simulink model "kopter_se_zavazim_Cascade_PID"  (R2024b)
settings: Solver=ode4  StartTime=0.0  StopTime=16  FixedStep=0.01  RelTol=1e-3
values from neighbouring files (symbols this model uses):
  A = 0.6081    [parametry_kopter_se_zavazim.m]
  b_moment = 3.6e-7    (= 3.6e-07)    [parametry_kopter_se_zavazim.m]
  d = 1    [parametry_kopter_se_zavazim.m]
  g = 9.81    [parametry_kopter_se_zavazim.m]
  Ip = m*d^2    (= 1)    [parametry_kopter_se_zavazim.m]
  Ixx = 0.0222    [parametry_kopter_se_zavazim.m]
  Iyy = 0.0222    [parametry_kopter_se_zavazim.m]
  Izz = 0.0429    [parametry_kopter_se_zavazim.m]
  k_thrust = 9.3e-6    (= 9.3e-06)    [parametry_kopter_se_zavazim.m]
  l = 0.2051    [parametry_kopter_se_zavazim.m]
  M = 2    [parametry_kopter_se_zavazim.m]
  m = 1    [parametry_kopter_se_zavazim.m]
  T = 0.8682    [parametry_kopter_se_zavazim.m]
  Us = [(M+m)*g; 0; 0; 0]    [parametry_kopter_se_zavazim.m]
  Xinit_ss = [Xinit_matrix; [0 0 0 0 0 0 0 0]']    [parametry_kopter_se_zavazim.m]
  Xs = [0;0;0; 0;0;0; 0;0; 0;0;0; 0;0;0; 0;0]    [parametry_kopter_se_zavazim.m]
undefined symbols (not defined in the file or in its folder): L, Us_p, Xs_p
libraries: simulink_extras x21, slpidlib x21, simulink x6
(part 2 of 5)

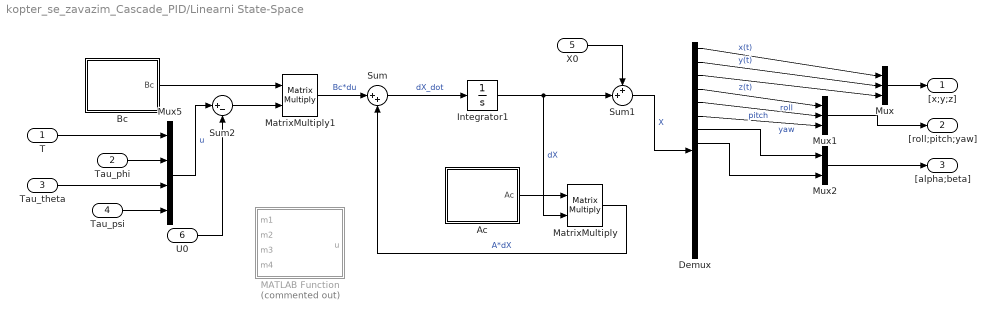
== system kopter_se_zavazim_Cascade_PID/Linearni State-Space ==
  T : Inport
  Tau_phi : Inport  Port=2
  Tau_theta : Inport  Port=3
  Tau_psi : Inport  Port=4
  X0 : Inport  Port=5
  U0 : Inport  Port=6
  Ac : MATLAB Function  TreatAsAtomicUnit=on
  Bc : MATLAB Function  TreatAsAtomicUnit=on
  Demux : Demux  Outputs=16
  Integrator1 : Integrator  InitialCondition=Xinit_ss - Xs
  MATLAB Function : MATLAB Function  Commented=on  TreatAsAtomicUnit=on
  MatrixMultiply : Product  Multiplication=Matrix(*)
  MatrixMultiply1 : Product  Multiplication=Matrix(*)
  Mux : Mux  Inputs=3
  Mux1 : Mux  Inputs=3
  Mux2 : Mux  Inputs=2
  Mux5 : Mux
  Sum : Sum  Inputs=|++
  Sum1 : Sum  Inputs=++|
  Sum2 : Sum  Inputs=|+-
  "[x;y;z]" : Outport
  "[roll;pitch;yaw]" : Outport  Port=2
  "[alpha;beta]" : Outport  Port=3
  wires:
  Ac/1(Ac) -> MatrixMultiply/1
  Integrator1/1 -> Sum1/2, MatrixMultiply/2  "dX"
  Demux/1 -> Mux/1  "x(t)"
  Demux/2 -> Mux/2  "y(t)"
  Demux/3 -> Mux/3  "z(t)"
  Mux/1 -> "[x;y;z]"/1
  Demux/4 -> Mux1/1  "roll"
  Demux/5 -> Mux1/2  "pitch"
  Demux/6 -> Mux1/3  "yaw"
  Mux1/1 -> "[roll;pitch;yaw]"/1
  Sum/1 -> Integrator1/1  "dX_dot"
  MatrixMultiply1/1 -> Sum/1  "Bc*du"
  MatrixMultiply/1 -> Sum/2  "A*dX"
  Bc/1(Bc) -> MatrixMultiply1/1
  Sum1/1 -> Demux/1  "X"
  Sum2/1 -> MatrixMultiply1/2
  Mux2/1 -> "[alpha;beta]"/1
  Demux/7 -> Mux2/1
  Demux/8 -> Mux2/2
  X0/1 -> Sum1/1
  U0/1 -> Sum2/2
  Mux5/1 -> Sum2/1  "u"
  Tau_psi/1 -> Mux5/4
  Tau_phi/1 -> Mux5/2
  Tau_theta/1 -> Mux5/3
  T/1 -> Mux5/1

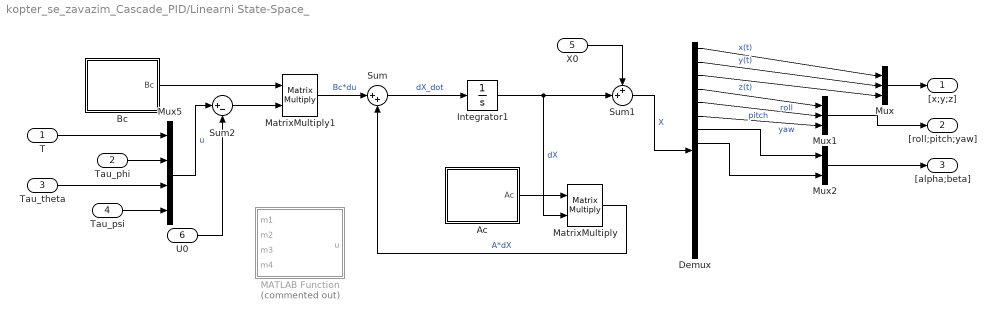
== system kopter_se_zavazim_Cascade_PID/Linearni State-Space_ ==
  T : Inport
  Tau_phi : Inport  Port=2
  Tau_theta : Inport  Port=3
  Tau_psi : Inport  Port=4
  X0 : Inport  Port=5
  U0 : Inport  Port=6
  Ac : MATLAB Function  TreatAsAtomicUnit=on
  Bc : MATLAB Function  TreatAsAtomicUnit=on
  Demux : Demux  Outputs=16
  Integrator1 : Integrator  InitialCondition=Xinit_ss
  MATLAB Function : MATLAB Function  Commented=on  TreatAsAtomicUnit=on
  MatrixMultiply : Product  Multiplication=Matrix(*)
  MatrixMultiply1 : Product  Multiplication=Matrix(*)
  Mux : Mux  Inputs=3
  Mux1 : Mux  Inputs=3
  Mux2 : Mux  Inputs=2
  Mux5 : Mux
  Sum : Sum  Inputs=|++
  Sum1 : Sum  Inputs=++|
  Sum2 : Sum  Inputs=|+-
  "[x;y;z]" : Outport
  "[roll;pitch;yaw]" : Outport  Port=2
  "[alpha;beta]" : Outport  Port=3
  wires:
  Ac/1(Ac) -> MatrixMultiply/1
  Integrator1/1 -> Sum1/2, MatrixMultiply/2  "dX"
  Demux/1 -> Mux/1  "x(t)"
  Demux/2 -> Mux/2  "y(t)"
  Demux/3 -> Mux/3  "z(t)"
  Mux/1 -> "[x;y;z]"/1
  Demux/4 -> Mux1/1  "roll"
  Demux/5 -> Mux1/2  "pitch"
  Demux/6 -> Mux1/3  "yaw"
  Mux1/1 -> "[roll;pitch;yaw]"/1
  Sum/1 -> Integrator1/1  "dX_dot"
  MatrixMultiply1/1 -> Sum/1  "Bc*du"
  MatrixMultiply/1 -> Sum/2  "A*dX"
  Bc/1(Bc) -> MatrixMultiply1/1
  Sum1/1 -> Demux/1  "X"
  Sum2/1 -> MatrixMultiply1/2
  Mux2/1 -> "[alpha;beta]"/1
  Demux/7 -> Mux2/1
  Demux/8 -> Mux2/2
  X0/1 -> Sum1/1
  U0/1 -> Sum2/2
  Mux5/1 -> Sum2/1  "u"
  Tau_psi/1 -> Mux5/4
  Tau_phi/1 -> Mux5/2
  Tau_theta/1 -> Mux5/3
  T/1 -> Mux5/1

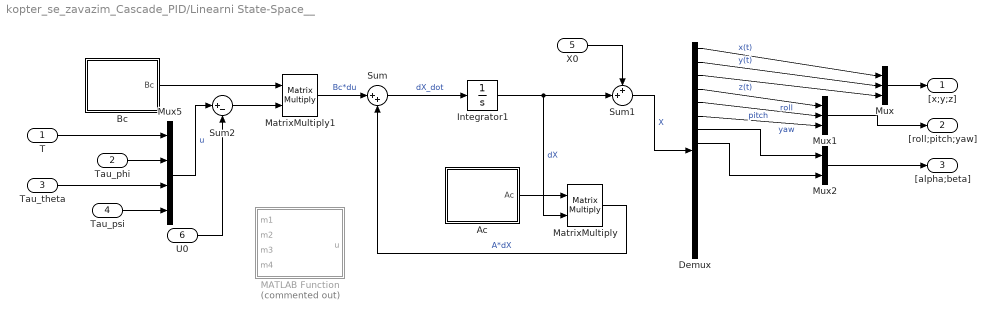
== system kopter_se_zavazim_Cascade_PID/Linearni State-Space__ ==
  T : Inport
  Tau_phi : Inport  Port=2
  Tau_theta : Inport  Port=3
  Tau_psi : Inport  Port=4
  X0 : Inport  Port=5
  U0 : Inport  Port=6
  Ac : MATLAB Function  TreatAsAtomicUnit=on
  Bc : MATLAB Function  TreatAsAtomicUnit=on
  Demux : Demux  Outputs=16
  Integrator1 : Integrator  InitialCondition=Xinit_ss
  MATLAB Function : MATLAB Function  Commented=on  TreatAsAtomicUnit=on
  MatrixMultiply : Product  Multiplication=Matrix(*)
  MatrixMultiply1 : Product  Multiplication=Matrix(*)
  Mux : Mux  Inputs=3
  Mux1 : Mux  Inputs=3
  Mux2 : Mux  Inputs=2
  Mux5 : Mux
  Sum : Sum  Inputs=|++
  Sum1 : Sum  Inputs=++|
  Sum2 : Sum  Inputs=|+-
  "[x;y;z]" : Outport
  "[roll;pitch;yaw]" : Outport  Port=2
  "[alpha;beta]" : Outport  Port=3
  wires:
  Ac/1(Ac) -> MatrixMultiply/1
  Integrator1/1 -> Sum1/2, MatrixMultiply/2  "dX"
  Demux/1 -> Mux/1  "x(t)"
  Demux/2 -> Mux/2  "y(t)"
  Demux/3 -> Mux/3  "z(t)"
  Mux/1 -> "[x;y;z]"/1
  Demux/4 -> Mux1/1  "roll"
  Demux/5 -> Mux1/2  "pitch"
  Demux/6 -> Mux1/3  "yaw"
  Mux1/1 -> "[roll;pitch;yaw]"/1
  Sum/1 -> Integrator1/1  "dX_dot"
  MatrixMultiply1/1 -> Sum/1  "Bc*du"
  MatrixMultiply/1 -> Sum/2  "A*dX"
  Bc/1(Bc) -> MatrixMultiply1/1
  Sum1/1 -> Demux/1  "X"
  Sum2/1 -> MatrixMultiply1/2
  Mux2/1 -> "[alpha;beta]"/1
  Demux/7 -> Mux2/1
  Demux/8 -> Mux2/2
  X0/1 -> Sum1/1
  U0/1 -> Sum2/2
  Mux5/1 -> Sum2/1  "u"
  Tau_psi/1 -> Mux5/4
  Tau_phi/1 -> Mux5/2
  Tau_theta/1 -> Mux5/3
  T/1 -> Mux5/1

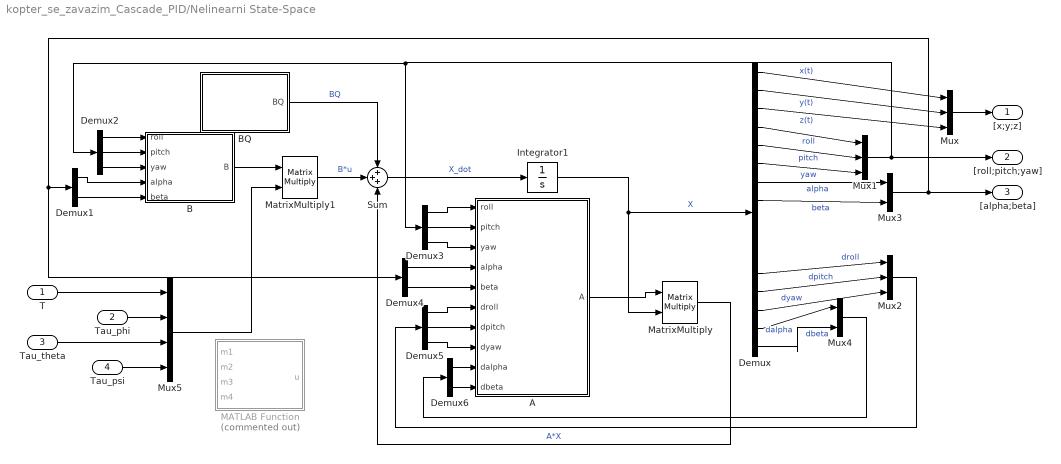
== system kopter_se_zavazim_Cascade_PID/Nelinearni State-Space ==
  T : Inport
  Tau_phi : Inport  Port=2
  Tau_theta : Inport  Port=3
  Tau_psi : Inport  Port=4
  A : MATLAB Function  TreatAsAtomicUnit=on
  B : MATLAB Function  TreatAsAtomicUnit=on
  BQ : MATLAB Function  TreatAsAtomicUnit=on
  Demux : Demux  Outputs=16
  Demux1 : Demux  Outputs=2
  Demux2 : Demux  Outputs=3
  Demux3 : Demux  Outputs=3
  Demux4 : Demux  Outputs=2
  Demux5 : Demux  Outputs=3
  Demux6 : Demux  Outputs=2
  Integrator1 : Integrator  InitialCondition=Xinit_ss
  MATLAB Function : MATLAB Function  Commented=on  TreatAsAtomicUnit=on
  MatrixMultiply : Product  Multiplication=Matrix(*)
  MatrixMultiply1 : Product  Multiplication=Matrix(*)
  Mux : Mux  Inputs=3
  Mux1 : Mux  Inputs=3
  Mux2 : Mux  Inputs=3
  Mux3 : Mux  Inputs=2
  Mux4 : Mux  Inputs=2
  Mux5 : Mux
  Sum : Sum  Inputs=+++
  "[x;y;z]" : Outport
  "[roll;pitch;yaw]" : Outport  Port=2
  "[alpha;beta]" : Outport  Port=3
  wires:
  A/1(A) -> MatrixMultiply/1
  Integrator1/1 -> MatrixMultiply/2, Demux/1  "X"
  Demux/1 -> Mux/1  "x(t)"
  Demux/2 -> Mux/2  "y(t)"
  Demux/3 -> Mux/3  "z(t)"
  Mux/1 -> "[x;y;z]"/1
  Demux/4 -> Mux1/1  "roll"
  Demux/5 -> Mux1/2  "pitch"
  Demux/6 -> Mux1/3  "yaw"
  Mux1/1 -> Demux2/1, Demux3/1, "[roll;pitch;yaw]"/1
  Demux/12 -> Mux2/1  "droll"
  Demux/13 -> Mux2/2  "dpitch"
  Demux/14 -> Mux2/3  "dyaw"
  Demux2/1 -> B/1(roll)
  Demux2/2 -> B/2(pitch)
  Demux2/3 -> B/3(yaw)
  Demux3/2 -> A/2(pitch)
  Demux3/1 -> A/1(roll)
  Demux3/3 -> A/3(yaw)
  Demux5/2 -> A/7(dpitch)
  Demux5/1 -> A/6(droll)
  Demux5/3 -> A/8(dyaw)
  Sum/1 -> Integrator1/1  "X_dot"
  BQ/1(BQ) -> Sum/1  "BQ"
  MatrixMultiply1/1 -> Sum/2  "B*u"
  B/1(B) -> MatrixMultiply1/1
  MatrixMultiply/1 -> Sum/3  "A*X"
  Mux2/1 -> Demux5/1
  Demux/7 -> Mux3/1  "alpha"
  Demux/8 -> Mux3/2  "beta"
  Mux3/1 -> Demux4/1, Demux1/1, "[alpha;beta]"/1
  Demux1/2 -> B/5(beta)
  Demux1/1 -> B/4(alpha)
  Demux4/2 -> A/5(beta)
  Demux4/1 -> A/4(alpha)
  Demux/15 -> Mux4/1  "dalpha"
  Demux/16 -> Mux4/2  "dbeta"
  Demux6/1 -> A/9(dalpha)
  Demux6/2 -> A/10(dbeta)
  Mux4/1 -> Demux6/1
  Tau_theta/1 -> Mux5/3
  Tau_psi/1 -> Mux5/4
  Tau_phi/1 -> Mux5/2
  Mux5/1 -> MatrixMultiply1/2
  T/1 -> Mux5/1

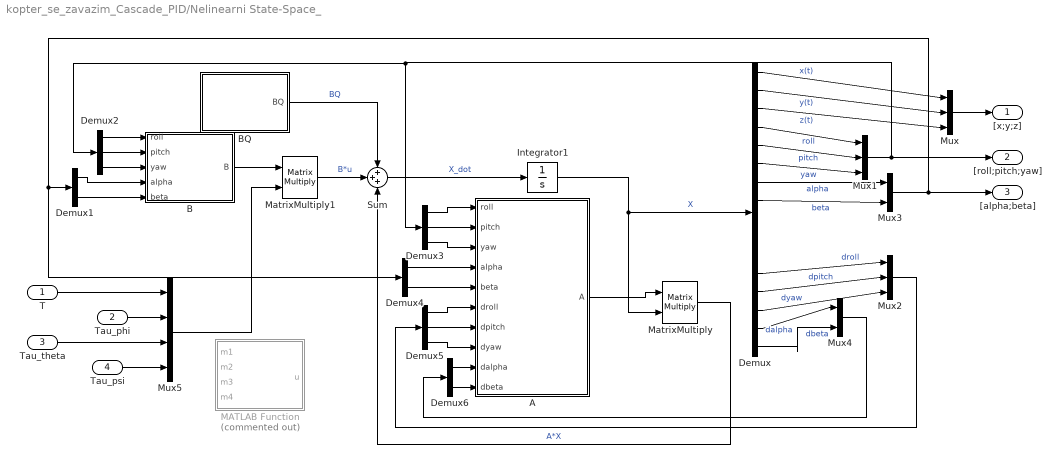
== system kopter_se_zavazim_Cascade_PID/Nelinearni State-Space_ ==
  T : Inport
  Tau_phi : Inport  Port=2
  Tau_theta : Inport  Port=3
  Tau_psi : Inport  Port=4
  A : MATLAB Function  TreatAsAtomicUnit=on
  B : MATLAB Function  TreatAsAtomicUnit=on
  BQ : MATLAB Function  TreatAsAtomicUnit=on
  Demux : Demux  Outputs=16
  Demux1 : Demux  Outputs=2
  Demux2 : Demux  Outputs=3
  Demux3 : Demux  Outputs=3
  Demux4 : Demux  Outputs=2
  Demux5 : Demux  Outputs=3
  Demux6 : Demux  Outputs=2
  Integrator1 : Integrator  InitialCondition=Xinit_ss
  MATLAB Function : MATLAB Function  Commented=on  TreatAsAtomicUnit=on
  MatrixMultiply : Product  Multiplication=Matrix(*)
  MatrixMultiply1 : Product  Multiplication=Matrix(*)
  Mux : Mux  Inputs=3
  Mux1 : Mux  Inputs=3
  Mux2 : Mux  Inputs=3
  Mux3 : Mux  Inputs=2
  Mux4 : Mux  Inputs=2
  Mux5 : Mux
  Sum : Sum  Inputs=+++
  "[x;y;z]" : Outport
  "[roll;pitch;yaw]" : Outport  Port=2
  "[alpha;beta]" : Outport  Port=3
  wires:
  A/1(A) -> MatrixMultiply/1
  Integrator1/1 -> MatrixMultiply/2, Demux/1  "X"
  Demux/1 -> Mux/1  "x(t)"
  Demux/2 -> Mux/2  "y(t)"
  Demux/3 -> Mux/3  "z(t)"
  Mux/1 -> "[x;y;z]"/1
  Demux/4 -> Mux1/1  "roll"
  Demux/5 -> Mux1/2  "pitch"
  Demux/6 -> Mux1/3  "yaw"
  Mux1/1 -> Demux2/1, Demux3/1, "[roll;pitch;yaw]"/1
  Demux/12 -> Mux2/1  "droll"
  Demux/13 -> Mux2/2  "dpitch"
  Demux/14 -> Mux2/3  "dyaw"
  Demux2/1 -> B/1(roll)
  Demux2/2 -> B/2(pitch)
  Demux2/3 -> B/3(yaw)
  Demux3/2 -> A/2(pitch)
  Demux3/1 -> A/1(roll)
  Demux3/3 -> A/3(yaw)
  Demux5/2 -> A/7(dpitch)
  Demux5/1 -> A/6(droll)
  Demux5/3 -> A/8(dyaw)
  Sum/1 -> Integrator1/1  "X_dot"
  BQ/1(BQ) -> Sum/1  "BQ"
  MatrixMultiply1/1 -> Sum/2  "B*u"
  B/1(B) -> MatrixMultiply1/1
  MatrixMultiply/1 -> Sum/3  "A*X"
  Mux2/1 -> Demux5/1
  Demux/7 -> Mux3/1  "alpha"
  Demux/8 -> Mux3/2  "beta"
  Mux3/1 -> Demux4/1, Demux1/1, "[alpha;beta]"/1
  Demux1/2 -> B/5(beta)
  Demux1/1 -> B/4(alpha)
  Demux4/2 -> A/5(beta)
  Demux4/1 -> A/4(alpha)
  Demux/15 -> Mux4/1  "dalpha"
  Demux/16 -> Mux4/2  "dbeta"
  Demux6/1 -> A/9(dalpha)
  Demux6/2 -> A/10(dbeta)
  Mux4/1 -> Demux6/1
  Tau_theta/1 -> Mux5/3
  Tau_psi/1 -> Mux5/4
  Tau_phi/1 -> Mux5/2
  Mux5/1 -> MatrixMultiply1/2
  T/1 -> Mux5/1

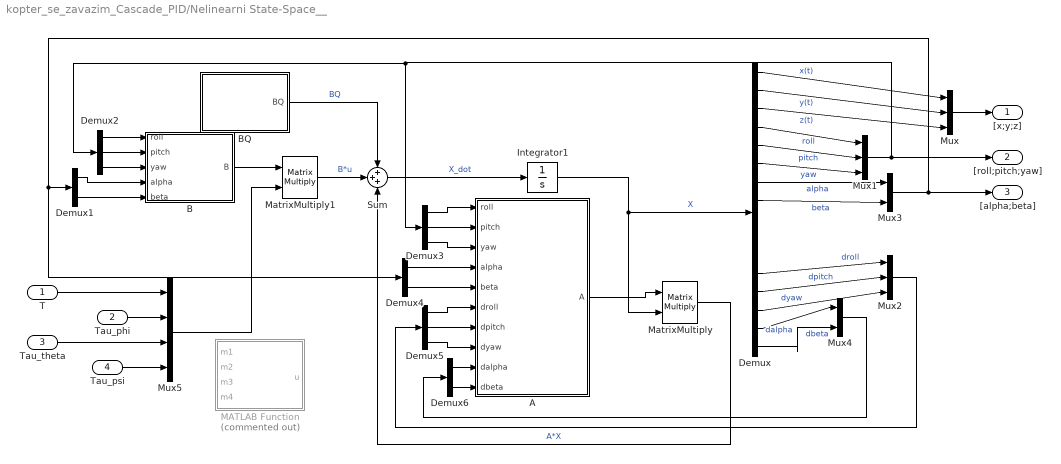
== system kopter_se_zavazim_Cascade_PID/Nelinearni State-Space__ ==
  T : Inport
  Tau_phi : Inport  Port=2
  Tau_theta : Inport  Port=3
  Tau_psi : Inport  Port=4
  A : MATLAB Function  TreatAsAtomicUnit=on
  B : MATLAB Function  TreatAsAtomicUnit=on
  BQ : MATLAB Function  TreatAsAtomicUnit=on
  Demux : Demux  Outputs=16
  Demux1 : Demux  Outputs=2
  Demux2 : Demux  Outputs=3
  Demux3 : Demux  Outputs=3
  Demux4 : Demux  Outputs=2
  Demux5 : Demux  Outputs=3
  Demux6 : Demux  Outputs=2
  Integrator1 : Integrator  InitialCondition=Xinit_ss
  MATLAB Function : MATLAB Function  Commented=on  TreatAsAtomicUnit=on
  MatrixMultiply : Product  Multiplication=Matrix(*)
  MatrixMultiply1 : Product  Multiplication=Matrix(*)
  Mux : Mux  Inputs=3
  Mux1 : Mux  Inputs=3
  Mux2 : Mux  Inputs=3
  Mux3 : Mux  Inputs=2
  Mux4 : Mux  Inputs=2
  Mux5 : Mux
  Sum : Sum  Inputs=+++
  "[x;y;z]" : Outport
  "[roll;pitch;yaw]" : Outport  Port=2
  "[alpha;beta]" : Outport  Port=3
  wires:
  A/1(A) -> MatrixMultiply/1
  Integrator1/1 -> MatrixMultiply/2, Demux/1  "X"
  Demux/1 -> Mux/1  "x(t)"
  Demux/2 -> Mux/2  "y(t)"
  Demux/3 -> Mux/3  "z(t)"
  Mux/1 -> "[x;y;z]"/1
  Demux/4 -> Mux1/1  "roll"
  Demux/5 -> Mux1/2  "pitch"
  Demux/6 -> Mux1/3  "yaw"
  Mux1/1 -> Demux2/1, Demux3/1, "[roll;pitch;yaw]"/1
  Demux/12 -> Mux2/1  "droll"
  Demux/13 -> Mux2/2  "dpitch"
  Demux/14 -> Mux2/3  "dyaw"
  Demux2/1 -> B/1(roll)
  Demux2/2 -> B/2(pitch)
  Demux2/3 -> B/3(yaw)
  Demux3/2 -> A/2(pitch)
  Demux3/1 -> A/1(roll)
  Demux3/3 -> A/3(yaw)
  Demux5/2 -> A/7(dpitch)
  Demux5/1 -> A/6(droll)
  Demux5/3 -> A/8(dyaw)
  Sum/1 -> Integrator1/1  "X_dot"
  BQ/1(BQ) -> Sum/1  "BQ"
  MatrixMultiply1/1 -> Sum/2  "B*u"
  B/1(B) -> MatrixMultiply1/1
  MatrixMultiply/1 -> Sum/3  "A*X"
  Mux2/1 -> Demux5/1
  Demux/7 -> Mux3/1  "alpha"
  Demux/8 -> Mux3/2  "beta"
  Mux3/1 -> Demux4/1, Demux1/1, "[alpha;beta]"/1
  Demux1/2 -> B/5(beta)
  Demux1/1 -> B/4(alpha)
  Demux4/2 -> A/5(beta)
  Demux4/1 -> A/4(alpha)
  Demux/15 -> Mux4/1  "dalpha"
  Demux/16 -> Mux4/2  "dbeta"
  Demux6/1 -> A/9(dalpha)
  Demux6/2 -> A/10(dbeta)
  Mux4/1 -> Demux6/1
  Tau_theta/1 -> Mux5/3
  Tau_psi/1 -> Mux5/4
  Tau_phi/1 -> Mux5/2
  Mux5/1 -> MatrixMultiply1/2
  T/1 -> Mux5/1

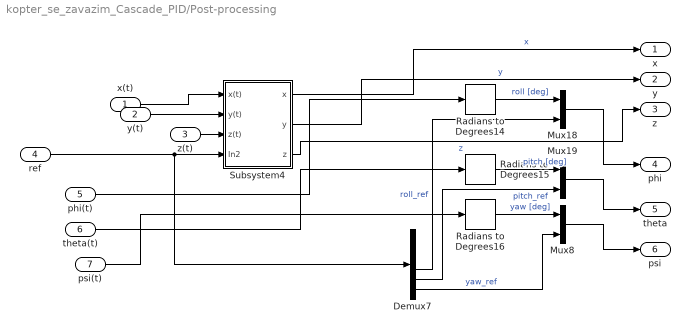
== system kopter_se_zavazim_Cascade_PID/Post-processing ==
  x(t) : Inport
  y(t) : Inport  Port=2
  z(t) : Inport  Port=3
  ref : Inport  Port=4
  phi(t) : Inport  Port=5
  theta(t) : Inport  Port=6
  psi(t) : Inport  Port=7
  Demux7 : Demux  Outputs=6
  Mux18 : Mux  Inputs=2
  Mux19 : Mux  Inputs=2
  Mux8 : Mux  Inputs=2
  Radians to Degrees14 : simulink_extras/Transformations/Radians to Degrees
  Radians to Degrees15 : simulink_extras/Transformations/Radians to Degrees
  Radians to Degrees16 : simulink_extras/Transformations/Radians to Degrees
  Subsystem4 : Subsystem
  x : Outport
  y : Outport  Port=2
  z : Outport  Port=3
  phi : Outport  Port=4
  theta : Outport  Port=5
  psi : Outport  Port=6
  wires:
  Radians to Degrees16/1 -> Mux8/1  "yaw [deg]"
  ref/1 -> Subsystem4/4(In2), Demux7/1
  Demux7/6 -> Mux8/2  "yaw_ref"
  theta(t)/1 -> Radians to Degrees15/1
  Demux7/4 -> Mux18/2  "roll_ref"
  Demux7/5 -> Mux19/2  "pitch_ref"
  Mux18/1 -> phi/1
  Subsystem4/3(z) -> z/1  "z"
  Radians to Degrees14/1 -> Mux18/1  "roll [deg]"
  Radians to Degrees15/1 -> Mux19/1  "pitch [deg]"
  Subsystem4/2(y) -> y/1  "y"
  x(t)/1 -> Subsystem4/1(x(t))
  y(t)/1 -> Subsystem4/2(y(t))
  psi(t)/1 -> Radians to Degrees16/1
  phi(t)/1 -> Radians to Degrees14/1
  Subsystem4/1(x) -> x/1  "x"
  Mux8/1 -> psi/1
  z(t)/1 -> Subsystem4/3(z(t))
  Mux19/1 -> theta/1

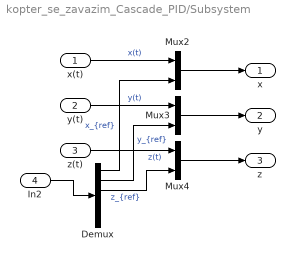
== system kopter_se_zavazim_Cascade_PID/Subsystem ==
  x(t) : Inport
  y(t) : Inport  Port=2
  z(t) : Inport  Port=3
  In2 : Inport  Port=4
  Demux : Demux  Outputs=6
  Mux2 : Mux  Inputs=2
  Mux3 : Mux  Inputs=2
  Mux4 : Mux  Inputs=2
  x : Outport
  y : Outport  Port=2
  z : Outport  Port=3
  wires:
  Demux/2 -> Mux3/2  "y_{ref}"
  Mux4/1 -> z/1
  y(t)/1 -> Mux3/1  "y(t)"
  Mux3/1 -> y/1
  Demux/1 -> Mux2/2  "x_{ref}"
  Demux/3 -> Mux4/2  "z_{ref}"
  Mux2/1 -> x/1
  In2/1 -> Demux/1
  x(t)/1 -> Mux2/1  "x(t)"
  z(t)/1 -> Mux4/1  "z(t)"

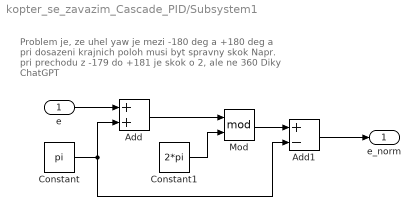
== system kopter_se_zavazim_Cascade_PID/Subsystem1 ==
  note: Problem je, ze uhel yaw je mezi -180 deg a +180 deg
      | a pri dosazeni krajnich poloh musi byt spravny skok
      | Napr. pri prechodu z -179 do +181 je skok o 2, ale ne 360
      | Diky ChatGPT
  e : Inport
  Add : Sum
  Add1 : Sum  Inputs=+-
  Constant : Constant  Value=pi
  Constant1 : Constant  Value=2*pi
  Mod : Math  Operator=mod
  e_norm : Outport
  wires:
  e/1 -> Add/1
  Add/1 -> Mod/1
  Constant/1 -> Add1/2, Add/2
  Constant1/1 -> Mod/2
  Mod/1 -> Add1/1
  Add1/1 -> e_norm/1

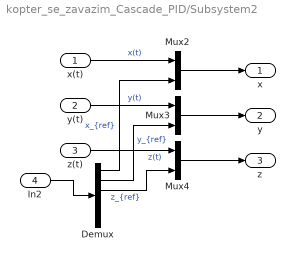
== system kopter_se_zavazim_Cascade_PID/Subsystem2 ==
  x(t) : Inport
  y(t) : Inport  Port=2
  z(t) : Inport  Port=3
  In2 : Inport  Port=4
  Demux : Demux  Outputs=6
  Mux2 : Mux  Inputs=2
  Mux3 : Mux  Inputs=2
  Mux4 : Mux  Inputs=2
  x : Outport
  y : Outport  Port=2
  z : Outport  Port=3
  wires:
  Demux/2 -> Mux3/2  "y_{ref}"
  Mux4/1 -> z/1
  y(t)/1 -> Mux3/1  "y(t)"
  Mux3/1 -> y/1
  Demux/1 -> Mux2/2  "x_{ref}"
  Demux/3 -> Mux4/2  "z_{ref}"
  Mux2/1 -> x/1
  In2/1 -> Demux/1
  x(t)/1 -> Mux2/1  "x(t)"
  z(t)/1 -> Mux4/1  "z(t)"

== system kopter_se_zavazim_Cascade_PID/Subsystem3 ==
  note: Problem je, ze uhel yaw je mezi -180 deg a +180 deg
      | a pri dosazeni krajnich poloh musi byt spravny skok
      | Napr. pri prechodu z -179 do +181 je skok o 2, ale ne 360
      | Diky ChatGPT
  e : Inport
  Add : Sum
  Add1 : Sum  Inputs=+-
  Constant : Constant  Value=pi
  Constant1 : Constant  Value=2*pi
  Mod : Math  Operator=mod
  e_norm : Outport
  wires:
  e/1 -> Add/1
  Add/1 -> Mod/1
  Constant/1 -> Add1/2, Add/2
  Constant1/1 -> Mod/2
  Mod/1 -> Add1/1
  Add1/1 -> e_norm/1

== system kopter_se_zavazim_Cascade_PID/[-pi; pi] calc ==
  note: Problem je, ze uhel yaw je mezi -180 deg a +180 deg
      | a pri dosazeni krajnich poloh musi byt spravny skok
      | Napr. pri prechodu z -179 do +181 je skok o 2, ale ne 360
      | Diky ChatGPT
  e : Inport
  Add : Sum
  Add1 : Sum  Inputs=+-
  Constant : Constant  Value=pi
  Constant1 : Constant  Value=2*pi
  Mod : Math  Operator=mod
  e_norm : Outport
  wires:
  e/1 -> Add/1
  Add/1 -> Mod/1
  Constant/1 -> Add1/2, Add/2
  Constant1/1 -> Mod/2
  Mod/1 -> Add1/1
  Add1/1 -> e_norm/1

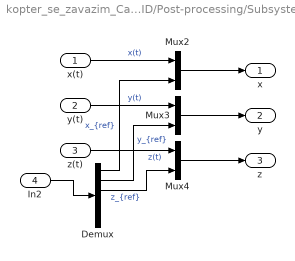
== system kopter_se_zavazim_Cascade_PID/Post-processing/Subsystem4 ==
  x(t) : Inport
  y(t) : Inport  Port=2
  z(t) : Inport  Port=3
  In2 : Inport  Port=4
  Demux : Demux  Outputs=6
  Mux2 : Mux  Inputs=2
  Mux3 : Mux  Inputs=2
  Mux4 : Mux  Inputs=2
  x : Outport
  y : Outport  Port=2
  z : Outport  Port=3
  wires:
  Demux/2 -> Mux3/2  "y_{ref}"
  Mux4/1 -> z/1
  y(t)/1 -> Mux3/1  "y(t)"
  Mux3/1 -> y/1
  Demux/1 -> Mux2/2  "x_{ref}"
  Demux/3 -> Mux4/2  "z_{ref}"
  Mux2/1 -> x/1
  In2/1 -> Demux/1
  x(t)/1 -> Mux2/1  "x(t)"
  z(t)/1 -> Mux4/1  "z(t)"

== matlab function kopter_se_zavazim_Cascade_PID/(rad//s)^2 na sily ==
  data: u output; U1 input; U2 input; U3 input; U4 input; k_thrust parameter; b_moment parameter; l parameter
function u = fcn(U1, U2, U3, U4, k_thrust, b_moment, l)

T = k_thrust*(U1+U2+U3+U4);
Tau_roll = k_thrust*l*(U1+U4-U2-U3);
Tau_pitch = k_thrust*l*(U3+U4-U1-U2);
Tau_yaw = b_moment*(U1+U3-U2-U4);

u = [T; Tau_roll; Tau_pitch; Tau_yaw];

== matlab function kopter_se_zavazim_Cascade_PID/Linearni State-Space_/Bc ==
  data: M parameter; Bc output; Ixx parameter; Iyy parameter; Izz parameter; m parameter
function Bc = fcn(M, Ixx, Iyy, Izz, m)
% Matice Bc linearizovana

Bc = [
        0,     0,     0,     0;
        0,     0,     0,     0;
        0,     0,     0,     0;
        0,     0,     0,     0;
        0,     0,     0,     0;
        0,     0,     0,     0;
        0,     0,     0,     0;
        0,     0,     0,     0;
        0,     0,     0,     0;
        0,     0,     0,     0;
1/(M + m),     0,     0,     0;
        0, 1/Ixx,     0,     0;
        0,     0, 1/Iyy,     0;
        0,     0,     0, 1/Izz;
        0,     0,     0,     0;
        0,     0,     0,     0];

== matlab function kopter_se_zavazim_Cascade_PID/Linearni State-Space_/MATLAB Function ==
  data: u output; m1 input; m2 input; m3 input; m4 input; k_thrust parameter; b_moment parameter; l parameter
function u = fcn(m1, m2, m3, m4, k_thrust, b_moment, l)

Thrust = k_thrust*(m1^2 + m2^2 + m3^2 + m4^2);
Tau_roll = l*k_thrust*(m1^2 + m4^2 - m2^2 - m3^2);
Tau_pitch = l*k_thrust*(m4^2 + m3^2 - m1^2 - m2^2);
Tau_yaw = b_moment*(m1^2 + m3^2 - m2^2 - m4^2);

u = [Thrust; Tau_roll; Tau_pitch; Tau_yaw];

== matlab function kopter_se_zavazim_Cascade_PID/Fi do [T; moments]_ ==
  data: F1 input; u output; F2 input; F3 input; F4 input; k_thrust parameter; b_moment parameter; l parameter
function u = fcn(F1, F2, F3, F4, k_thrust, b_moment, l)
% Dle X tvaru kvadrokoptery dopocitavam 
% celkovou tahovou silu T a tri momenty
T = F1+F2+F3+F4;
Tau_phi = l*(F1+F4-F2-F3);
Tau_theta = l*(F3+F4-F1-F2);
Tau_psi = b_moment/k_thrust*(F1-F2+F3-F4);

u = [T; Tau_phi; Tau_theta; Tau_psi];

== matlab function kopter_se_zavazim_Cascade_PID/Fi to [T; moments] ==
  data: F1 input; inputs output; F2 input; F3 input; F4 input; k_thrust parameter; b_moment parameter; l parameter
function inputs = fcn(F1, F2, F3, F4, k_thrust, b_moment, l)
% Dle X tvaru kvadrokoptery dopocitavam 
% celkovou tahovou silu T a tri momenty
T = F1+F2+F3+F4;
Tau_phi = l*(F1+F4-F2-F3);
Tau_theta = l*(F3+F4-F1-F2);
Tau_psi = b_moment/k_thrust*(F1-F2+F3-F4);

inputs = [T; Tau_phi; Tau_theta; Tau_psi];

== matlab function kopter_se_zavazim_Cascade_PID/Nelinearni State-Space_/A ==
  data: roll input; A output; pitch input; yaw input; alpha input; beta input; droll input; dpitch input; dyaw input; dalpha input; dbeta input; Ixx parameter; Iyy parameter; Izz parameter; M parameter; Ip parameter; d parameter; m parameter
function A = fcn(roll, pitch, yaw, alpha, beta, droll, dpitch, dyaw, dalpha, dbeta, Ixx, Iyy, Izz, M, Ip, d, m)
% Matice dynamiky A

phi_t = roll;
theta_t = pitch;
psi_t = yaw;

alpha_t = alpha;
beta_t = beta;

phi_dot_t = droll;
theta_dot_t = dpitch;
psi_dot_t = dyaw;

alpha_dot_t = dalpha;
beta_dot_t = dbeta;

A = [ 
0, 0, 0, 0, 0, 0, 0, 0, 1, 0, 0,                                                                                                                                                                                                                                                                                                                                                                                                                                                                                                           0,                                                                                                                                                                                                                                                                                                                                                                                                                                                                                                                                                                                                                                                                                                                              0,                                                                                                                                                                                            0,                                                          0,                                                  0;
0, 0, 0, 0, 0, 0, 0, 0, 0, 1, 0,                                                                                                                                                                                                                                                                                                                                                                                                                                                                                                           0,                                                                                                                                                                                                                                                                                                                                                                                                                                                                                                                                                                                                                                                                                                                              0,                                                                                                                                                                                            0,                                                          0,                                                  0;
0, 0, 0, 0, 0, 0, 0, 0, 0, 0, 1,                                                                                                                                                                                                                                                                                                                                                                                                                                                                                                           0,                                                                                                                                                                                                                                                                                                                                                                                                                                                                                                                                                                                                                                                                                                                              0,                                                                                                                                                                                            0,                                                          0,                                                  0;
0, 0, 0, 0, 0, 0, 0, 0, 0, 0, 0,                                                                                                                                                                                                                                                                                                                                                                                                                                                                                                           1,                                                                                                                                                                                                                                                                                                                                                                                                                                                                                                                                                                                                                                                                                                                              0,                                                                                                                                                                                            0,                                                          0,                                                  0;
0, 0, 0, 0, 0, 0, 0, 0, 0, 0, 0,                                                                                                                                                                                                                                                                                                                                                                                                                                                                                                           0,                                                                                                                                                                                                                                                                                                                                                                                                                                                                                                                                                                                                                                                                                                                              1,                                                                                                                                                                                            0,                                                          0,                                                  0;
0, 0, 0, 0, 0, 0, 0, 0, 0, 0, 0,                                                                                                                                                                                                                                                                                                                                                                                                                                                                                                           0,                                                                                                                                                                                                                                                                                                                                                                                                                                                                                                                                                                                                                                                                                                                              0,                                                                                                                                                                                            1,                                                          0,                                                  0;
0, 0, 0, 0, 0, 0, 0, 0, 0, 0, 0,                                                                                                                                                                                                                                                                                                                                                                                                                                                                                                           0,                                                                                                                                                                                                                                                                                                                                                                                                                                                                                                                                                                                                                                                                                                                              0,                                                                                                                                                                                            0,                                                          1,                                                  0;
0, 0, 0, 0, 0, 0, 0, 0, 0, 0, 0,                                                                                                                                                                                                                                                                                                                                                                                                                                                                                                           0,                                                                                                                                                                                                                                                                                                                                                                                                                                                                                                                                                                                                                                                                                                                              0,                                                                                                                                                                                            0,                                                          0,                                                  1;
0, 0, 0, 0, 0, 0, 0, 0, 0, 0, 0,                                                                                                                                                                                                                                                                                                                                                                                                                                                                                                           0,                                                                                                                                                                                                                                                                                                                                                                                                                                                                                                                                                                                                                                                                                                                              0,                                                                                                                                                                                            0,       (alpha_dot_t*d*m*cos(beta_t)^3*sin(alpha_t))/(M + m),  (beta_dot_t*d*m*cos(beta_t)*sin(alpha_t))/(M + m);
0, 0, 0, 0, 0, 0, 0, 0, 0, 0, 0,                                                                                                                                                                                                                                                                                                                                                                                                                                                                                                           0,                                                                                                                                                                                                                                                                                                                                                                                                                                                                                                                                                                                                                                                                                                                              0,                                                                                                                                                                                            0, -(alpha_dot_t*d*m*sin(beta_t)*(sin(beta_t)^2 - 1))/(M + m),               (beta_dot_t*d*m*sin(beta_t))/(M + m);
0, 0, 0, 0, 0, 0, 0, 0, 0, 0, 0,                                                                                                                                                                                                                                                                                                                                                                                                                                                                                                           0,                                                                                                                                                                                                                                                                                                                                                                                                                                                                                                                                                                                                                                                                                                                              0,                                                                                                                                                                                            0,      -(alpha_dot_t*d*m*cos(alpha_t)*cos(beta_t)^3)/(M + m), -(beta_dot_t*d*m*cos(alpha_t)*cos(beta_t))/(M + m);
0, 0, 0, 0, 0, 0, 0, 0, 0, 0, 0,                                       (sin(theta_t)*(Ixx*Izz*theta_dot_t - Izz^2*theta_dot_t + Iyy*Izz*theta_dot_t - Iyy^2*theta_dot_t*cos(phi_t)^2 + Izz^2*theta_dot_t*cos(phi_t)^2 + Ixx*Iyy*theta_dot_t*cos(phi_t)^2 - Ixx*Izz*theta_dot_t*cos(phi_t)^2 - Iyy^2*psi_dot_t*cos(phi_t)*cos(theta_t)*sin(phi_t) + Izz^2*psi_dot_t*cos(phi_t)*cos(theta_t)*sin(phi_t) + Ixx*Iyy*psi_dot_t*cos(phi_t)*cos(theta_t)*sin(phi_t) - Ixx*Izz*psi_dot_t*cos(phi_t)*cos(theta_t)*sin(phi_t)))/(Iyy*Izz*cos(theta_t)), - ((Iyy*Izz + Ixx*Iyy*sin(theta_t)^2 - Iyy*Izz*sin(theta_t)^2 - Ixx*Iyy*sin(phi_t)^2*sin(theta_t)^2 + Ixx*Izz*sin(phi_t)^2*sin(theta_t)^2)*((Izz*theta_dot_t*sin(2*phi_t))/2 - (Iyy*theta_dot_t*sin(2*phi_t))/2 + Ixx*psi_dot_t*cos(theta_t) - Iyy*psi_dot_t*cos(theta_t) + Izz*psi_dot_t*cos(theta_t) + 2*Iyy*psi_dot_t*cos(phi_t)^2*cos(theta_t) - 2*Izz*psi_dot_t*cos(phi_t)^2*cos(theta_t)))/(Ixx*Iyy*Izz*(sin(theta_t)^2 - 1)) - (sin(theta_t)^2*(Iyy - Iyy*sin(phi_t)^2 + Izz*sin(phi_t)^2)*((Iyy*theta_dot_t*sin(2*phi_t))/2 - (Izz*theta_dot_t*sin(2*phi_t))/2 - 2*Ixx*psi_dot_t*cos(theta_t) + 2*Izz*psi_dot_t*cos(phi_t)^2*cos(theta_t) + 2*Iyy*psi_dot_t*cos(theta_t)*sin(phi_t)^2))/(Iyy*Izz*(sin(theta_t)^2 - 1)), (psi_dot_t*sin(2*phi_t)*(Iyy - Izz)*(Ixx^2*cos(2*theta_t) - Ixx^2 + Ixx*Iyy + Ixx*Izz + Iyy*Izz - Ixx*Iyy*cos(2*theta_t) - Ixx*Izz*cos(2*theta_t) + Iyy*Izz*cos(2*theta_t)))/(4*Ixx*Iyy*Izz),                                                          0,                                                  0;
0, 0, 0, 0, 0, 0, 0, 0, 0, 0, 0, -(Izz^2*theta_dot_t*sin(2*phi_t) - Izz^2*psi_dot_t*cos(theta_t) - Iyy^2*theta_dot_t*sin(2*phi_t) - Iyy^2*psi_dot_t*cos(theta_t) + Ixx*Iyy*psi_dot_t*cos(theta_t) + Ixx*Izz*psi_dot_t*cos(theta_t) + 2*Iyy*Izz*psi_dot_t*cos(theta_t) + Iyy^2*psi_dot_t*cos(2*phi_t)*cos(theta_t) - Izz^2*psi_dot_t*cos(2*phi_t)*cos(theta_t) + Ixx*Iyy*theta_dot_t*sin(2*phi_t) - Ixx*Izz*theta_dot_t*sin(2*phi_t) - Ixx*Iyy*psi_dot_t*cos(2*phi_t)*cos(theta_t) + Ixx*Izz*psi_dot_t*cos(2*phi_t)*cos(theta_t))/(2*Iyy*Izz),                                                                                                                                                                                                                                                                                                                                                                                                                                                                                                                                                                                                                                        -(psi_dot_t*cos(phi_t)*sin(phi_t)*sin(theta_t)*(Iyy - Izz)*(Iyy - Ixx + Izz))/(Iyy*Izz),                           (psi_dot_t*sin(2*theta_t)*(Iyy^2*cos(2*phi_t) - Izz^2*cos(2*phi_t) - Iyy^2 - Izz^2 + Ixx*Iyy + Ixx*Izz - Ixx*Iyy*cos(2*phi_t) + Ixx*Izz*cos(2*phi_t)))/(4*Iyy*Izz),                                                          0,                                                  0;
0, 0, 0, 0, 0, 0, 0, 0, 0, 0, 0,                                            (Ixx*Iyy*theta_dot_t - Izz^2*theta_dot_t - Iyy^2*theta_dot_t + Ixx*Izz*theta_dot_t + 2*Iyy*Izz*theta_dot_t - Iyy^2*theta_dot_t*cos(2*phi_t) + Izz^2*theta_dot_t*cos(2*phi_t) - Iyy^2*psi_dot_t*sin(2*phi_t)*cos(theta_t) + Izz^2*psi_dot_t*sin(2*phi_t)*cos(theta_t) + Ixx*Iyy*theta_dot_t*cos(2*phi_t) - Ixx*Izz*theta_dot_t*cos(2*phi_t) + Ixx*Iyy*psi_dot_t*sin(2*phi_t)*cos(theta_t) - Ixx*Izz*psi_dot_t*sin(2*phi_t)*cos(theta_t))/(2*Iyy*Izz*cos(theta_t)),                                                                                                                                                                                                                                                                                                                                                                                                                                                                                                                                                                                                                  (psi_dot_t*sin(theta_t)*(Iyy - Iyy*sin(phi_t)^2 + Izz*sin(phi_t)^2)*(Iyy - Ixx + Izz))/(Iyy*Izz*cos(theta_t)),                                                                                                       (psi_dot_t*cos(phi_t)*sin(phi_t)*sin(theta_t)*(Iyy - Izz)*(Iyy - Ixx + Izz))/(Iyy*Izz),                                                          0,                                                  0;
0, 0, 0, 0, 0, 0, 0, 0, 0, 0, 0,                                                                                                                                                                                                                                                                                                                                                                                                                                                                                                           0,                                                                                                                                                                                                                                                                                                                                                                                                                                                                                                                                                                                                                                                                                                                              0,                                                                                                                                                                                            0,                     (2*beta_dot_t*sin(beta_t))/cos(beta_t),                                                  0;
0, 0, 0, 0, 0, 0, 0, 0, 0, 0, 0,                                                                                                                                                                                                                                                                                                                                                                                                                                                                                                           0,                                                                                                                                                                                                                                                                                                                                                                                                                                                                                                                                                                                                                                                                                                                              0,                                                                                                                                                                                            0,                             -(alpha_dot_t*sin(2*beta_t))/2,                                                  0];
